simulink model "SiDrivetrain"  (R2019b)
settings: Solver=ode23tb  StartTime=0.0  StopTime=50  RelTol=1e-3  EnableMultiTasking=on
model workspace (MAT data in the model file):
  N = [-4.7 4.75 4.75 3.75 3.25 2.75 2.25 1.5 1 0.75]
  NF : Simulink.Parameter (value not decoded)
  NR : Simulink.Parameter (value not decoded)
  Ndiff = 3
  RWheel = 0.3
  b_axle : Simulink.Parameter (value not decoded)
  b_driveshaft : Simulink.Parameter (value not decoded)
  dt_DCT : Simulink.Parameter (value not decoded)
  k_axle : Simulink.Parameter (value not decoded)
  k_driveshaft : Simulink.Parameter (value not decoded)
  k_hyd : Simulink.Parameter (value not decoded)
  tau_hyd : Simulink.Parameter (value not decoded)
  wc_shaft : Simulink.Parameter (value not decoded)
values from neighbouring files (symbols this model uses):
  b_axle = 10.0    [DrivetrainEvDD.sldd]    (also in DrivetrainHevMmDD.sldd; SiDrivetrainDD.sldd)
  b_driveshaft = 10.0    [DrivetrainEvDD.sldd]    (also in DrivetrainHevMmDD.sldd; SiDrivetrainDD.sldd)
  k_axle = 5000.0    [DrivetrainEvDD.sldd]    (also in DrivetrainHevMmDD.sldd; SiDrivetrainDD.sldd)
  k_driveshaft = 1000.0    [DrivetrainEvDD.sldd]    (also in DrivetrainHevMmDD.sldd; SiDrivetrainDD.sldd)
symbols that are objects in the model workspace (value not decoded): k_hyd, tau_hyd
libraries: autolibsharedcoupling x12, autolibpowerinfoutils x6, autolibshareddiff x4, autolibutils x3, autolibshared x3, autolibcoupling x2, simulink x2, autolibsharedtransfixedgear x2, autolibtransdct x1, autolibshareddrivetraincommon x1, autolibtranscontrols x1
(part 4 of 4)

== system SiDrivetrain/Differential and Compliance/Front Wheel Drive/Front Axle Compliance 2 ==
  Info : Inport
  Bus Selector : BusSelector  OutputSignals=PwrInfo.PwrTrnsfrd,PwrInfo.PwrNotTrnsfrd,PwrInfo.PwrStored
  Bus Selector1 : BusSelector  OutputSignals=Trq.R,Trq.C
  Power Accounting Bus Creator : autolibpowerinfoutils/Power Accounting Bus Creator  AssctBlkSelPopup=Parent  RefBlkName='libraryname/blkname'  PwrTrnsfrdCheckBox=on  PwrNotTrnsfrdCheckBox=on  PwrStoredCheckBox=on  aMode=aMode
      settings: SourceProductName=Powertrain Blockset  SourceProductBaseCode=PW
  Terminator : Terminator
  Terminator1 : Terminator
  Terminator2 : Terminator
  Two-Way Connection1 : TwoWayConnection
  Two-Way Connection4 : TwoWayConnection
  R : PMIOPort  Side=Left
  C : PMIOPort  Port=2  Side=Right
  wires:
  Two-Way Connection4/1 -> Terminator/1
  Info/1 -> Bus Selector1/1, Bus Selector/1
  Two-Way Connection1/1 -> Terminator1/1
  Bus Selector1/1 -> Two-Way Connection4/1  "<R>"
  Bus Selector1/2 -> Two-Way Connection1/1  "<C>"
  Power Accounting Bus Creator/1 -> Terminator2/1
  Bus Selector/1 -> Power Accounting Bus Creator/1  "<PwrTrnsfrd>"
  Bus Selector/2 -> Power Accounting Bus Creator/2  "<PwrNotTrnsfrd>"
  Bus Selector/3 -> Power Accounting Bus Creator/3  "<PwrStored>"
  connections:
  R/RConn1 -- Two-Way Connection4/RConn1
  Two-Way Connection1/RConn1 -- C/RConn1

== system SiDrivetrain/Differential and Compliance/Front Wheel Drive/Rear Axle 1 ==
  Ground : Ground
  Terminator1 : Terminator
  Two-Way Connection : TwoWayConnection
  RA1 : PMIOPort  Side=Right
  wires:
  Two-Way Connection/1 -> Terminator1/1
  Ground/1 -> Two-Way Connection/1
  connections:
  Two-Way Connection/RConn1 -- RA1/RConn1

== system SiDrivetrain/Differential and Compliance/Front Wheel Drive/Rear Axle 2 ==
  Ground1 : Ground
  Terminator : Terminator
  Two-Way Connection4 : TwoWayConnection
  RA2 : PMIOPort  Side=Right
  wires:
  Two-Way Connection4/1 -> Terminator/1
  Ground1/1 -> Two-Way Connection4/1
  connections:
  Two-Way Connection4/RConn1 -- RA2/RConn1

== system SiDrivetrain/Differential and Compliance/Rear Wheel Drive/Front Axle 1 ==
  Ground : Ground
  Terminator1 : Terminator
  Two-Way Connection : TwoWayConnection
  FA1 : PMIOPort  Side=Right
  wires:
  Two-Way Connection/1 -> Terminator1/1
  Ground/1 -> Two-Way Connection/1
  connections:
  Two-Way Connection/RConn1 -- FA1/RConn1

== system SiDrivetrain/Differential and Compliance/Rear Wheel Drive/Front Axle 2 ==
  Ground1 : Ground
  Terminator : Terminator
  Two-Way Connection4 : TwoWayConnection
  FA2 : PMIOPort  Side=Right
  wires:
  Two-Way Connection4/1 -> Terminator/1
  Ground1/1 -> Two-Way Connection4/1
  connections:
  Two-Way Connection4/RConn1 -- FA2/RConn1

== system SiDrivetrain/Differential and Compliance/Rear Wheel Drive/Rear Axle Compliance 2 ==
  Info : Inport
  Bus Selector : BusSelector  OutputSignals=PwrInfo.PwrTrnsfrd,PwrInfo.PwrNotTrnsfrd,PwrInfo.PwrStored
  Bus Selector1 : BusSelector  OutputSignals=Trq.R,Trq.C
  Power Accounting Bus Creator : autolibpowerinfoutils/Power Accounting Bus Creator  AssctBlkSelPopup=Parent  RefBlkName='libraryname/blkname'  PwrTrnsfrdCheckBox=on  PwrNotTrnsfrdCheckBox=on  PwrStoredCheckBox=on  aMode=aMode
      settings: SourceProductName=Powertrain Blockset  SourceProductBaseCode=PW
  Terminator : Terminator
  Terminator1 : Terminator
  Terminator2 : Terminator
  Two-Way Connection1 : TwoWayConnection
  Two-Way Connection4 : TwoWayConnection
  R : PMIOPort  Side=Left
  C : PMIOPort  Port=2  Side=Right
  wires:
  Two-Way Connection4/1 -> Terminator/1
  Info/1 -> Bus Selector1/1, Bus Selector/1
  Two-Way Connection1/1 -> Terminator1/1
  Bus Selector1/1 -> Two-Way Connection4/1  "<R>"
  Bus Selector1/2 -> Two-Way Connection1/1  "<C>"
  Power Accounting Bus Creator/1 -> Terminator2/1
  Bus Selector/1 -> Power Accounting Bus Creator/1  "<PwrTrnsfrd>"
  Bus Selector/2 -> Power Accounting Bus Creator/2  "<PwrNotTrnsfrd>"
  Bus Selector/3 -> Power Accounting Bus Creator/3  "<PwrStored>"
  connections:
  R/RConn1 -- Two-Way Connection4/RConn1
  Two-Way Connection1/RConn1 -- C/RConn1

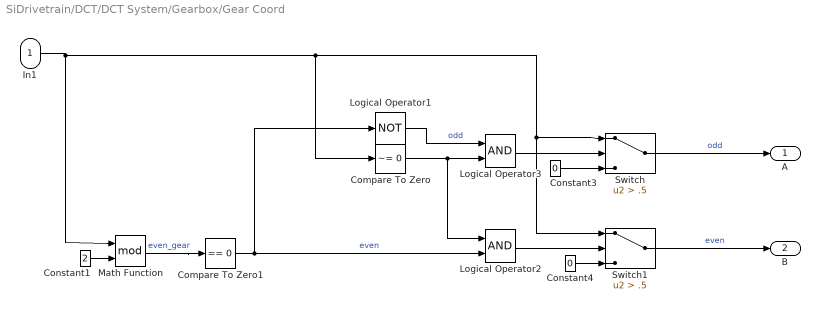
== system SiDrivetrain/DCT/DCT System/Gearbox/Gear Coord ==
  In1 : Inport
  Compare To Zero : simulink/Logic and Bit Operations/Compare To Zero  relop=~=  OutDataTypeStr=boolean
  Compare To Zero1 : simulink/Logic and Bit Operations/Compare To Zero  relop===  OutDataTypeStr=boolean
  Constant1 : Constant  Value=2
  Constant3 : Constant  Value=0
  Constant4 : Constant  Value=0
  Logical Operator1 : Logic  Operator=NOT  AllPortsSameDT=off  OutDataTypeStr=boolean
  Logical Operator2 : Logic  AllPortsSameDT=off  OutDataTypeStr=boolean
  Logical Operator3 : Logic  AllPortsSameDT=off  OutDataTypeStr=boolean
  Math Function : Math  Operator=mod  SaturateOnIntegerOverflow=on
  Switch : Switch  Criteria=u2 > Threshold  Threshold=.5
  Switch1 : Switch  Criteria=u2 > Threshold  Threshold=.5
  A : Outport  VectorParamsAs1DForOutWhenUnconnected=off
  B : Outport  Port=2  VectorParamsAs1DForOutWhenUnconnected=off
  wires:
  In1/1 -> Switch/1, Switch1/1, Compare To Zero/1, Math Function/1
  Math Function/1 -> Compare To Zero1/1  "even_gear"
  Constant1/1 -> Math Function/2
  Compare To Zero1/1 -> Logical Operator1/1, Logical Operator2/2  "even"
  Constant4/1 -> Switch1/3
  Switch/1 -> A/1  "odd"
  Constant3/1 -> Switch/3
  Switch1/1 -> B/1  "even"
  Logical Operator2/1 -> Switch1/2
  Logical Operator3/1 -> Switch/2
  Compare To Zero/1 -> Logical Operator2/1, Logical Operator3/2
  Logical Operator1/1 -> Logical Operator3/1  "odd"

== system SiDrivetrain/DCT/DCT System/Hydraulics/A Hydraulics Tau ==
  In1 : Inport
  In2 : Inport  Port=2
  2*pi : Gain  Gain=2*pi
  ClutchGain : Gain  Gain=k_hyd
  Constant1 : Constant  Value=0
  Constant2 : Constant  Value=tau_hyd
  Cont LPF Dyn : autolibutils/Cont LPF Dyn  aMode=aMode  dataType=off
      settings: SourceProductName=Powertrain Blockset  SourceProductBaseCode=PW
  Product : Product  Inputs=/
  Switch : Switch  Criteria=u2 ~= 0
  Out1 : Outport  VectorParamsAs1DForOutWhenUnconnected=off
  wires:
  In1/1 -> Switch/2
  ClutchGain/1 -> Out1/1
  Constant2/1 -> Product/1
  Cont LPF Dyn/1 -> ClutchGain/1
  Switch/1 -> Cont LPF Dyn/1
  Product/1 -> 2*pi/1
  In2/1 -> Switch/1
  2*pi/1 -> Cont LPF Dyn/2
  Constant1/1 -> Switch/3

== system SiDrivetrain/DCT/DCT System/Hydraulics/B Hydraulics Tau ==
  In1 : Inport
  In2 : Inport  Port=2
  2*pi : Gain  Gain=2*pi
  ClutchGain : Gain  Gain=k_hyd
  Constant1 : Constant  Value=0
  Constant2 : Constant  Value=tau_hyd
  Cont LPF Dyn : autolibutils/Cont LPF Dyn  aMode=aMode  dataType=off
      settings: SourceProductName=Powertrain Blockset  SourceProductBaseCode=PW
  Product : Product  Inputs=/
  Switch : Switch  Criteria=u2 ~= 0
  Out1 : Outport  VectorParamsAs1DForOutWhenUnconnected=off
  wires:
  Constant1/1 -> Switch/3
  2*pi/1 -> Cont LPF Dyn/2
  In2/1 -> Switch/1
  Product/1 -> 2*pi/1
  Switch/1 -> Cont LPF Dyn/1
  Cont LPF Dyn/1 -> ClutchGain/1
  Constant2/1 -> Product/1
  ClutchGain/1 -> Out1/1
  In1/1 -> Switch/2
